simulink library "Suspension"  (R2025b)
settings: Solver=VariableStepAuto  StartTime=0.0  StopTime=10.0  RelTol=1e-3
undefined symbols (not defined in the file): Init, Vehicle
libraries: Susp_AxleTA2PR x1, Susp_AxleTA3 x1, Susp_AxleTA4Watts x1, Susp_LUT x1, Suspension_Linkage x1, Suspension_Linkage_Decoupled x1, Susp_LiveAxle x1, Susp_DOF15 x1, Susp_TwistBeam x1
Description:
  | Component of Simscape Vehicle Templates Library
  | 
  | Copyright 2018-2025 The MathWorks, Inc.
settings Model: Creator=smiller  LastModifiedBy=smiller
settings SolverCC: AlgebraicLoopSolver=TrustRegion
settings DataIOCC: ReturnWorkspaceOutputs=off
settings DebuggingCC: UnconnectedInputMsg=warning  UnconnectedOutputMsg=warning  UnconnectedLineMsg=warning  ArithmeticOperatorsInVariantConditions=warning
settings ModelReferenceCC: EnableRefExpFcnMdlSchedulingChecks=on
settings SFSimCC: CustomCodeUndefinedFunction=UseInterfaceOnly
settings RTWCC: GPUComputeCapability=3.5

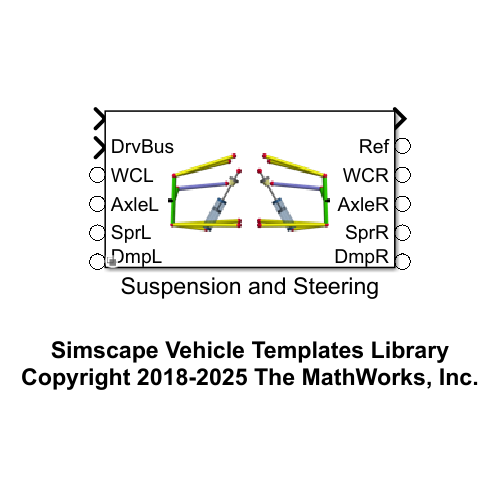
[thumbnail: Simulink's stored preview of the top-level diagram]
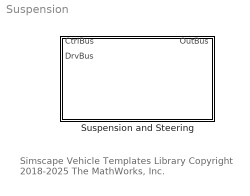
== system Suspension ==
  note: Simscape Vehicle Templates Library
      | Copyright 2018-2025 The MathWorks, Inc.
  Suspension and Steering : Subsystem  Variant=on  VariantControlMode=label  VariantControl=Variant1  LabelModeActiveChoice=Linkage  mask(Suspension and Steering){Susp=Vehicle.Chassis.SuspA1, Init=Init.Axle1, VariantLabel=Vehicle.Chassis.SuspA1.class.Value}
      mask prompts: Susp "Suspension Parameters"; Init "Initial Values"; VariantLabel "Variant Label"
      mask help: Models suspension and optional steering system for one axle. Option is chosen by string provided in Variant Label. The parameters for the selected option are contained in Suspension Parameters data structure.
      mask init:
      | curblk = gcb;
      | 
      | % Set variant for this block 
      | set_param(curblk,'LabelModeActiveChoice',VariantLabel);

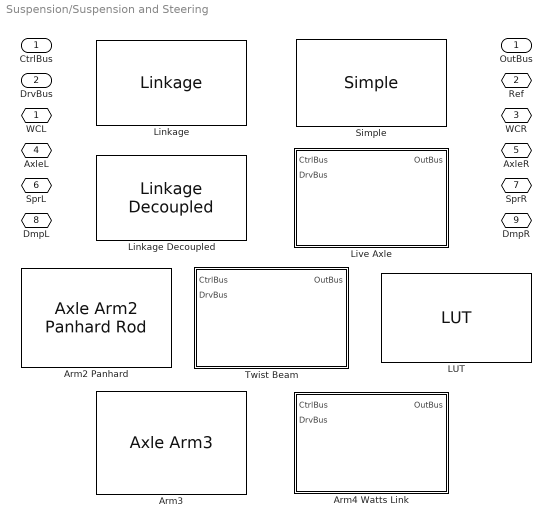
== system Suspension/Suspension and Steering ==
  "CtrlBus " : Inport
  DrvBus : Inport  Port=2
  Arm2 Panhard : Susp_AxleTA2PR/Axle Arm2 Panhard Rod  VariantControl=AxleTA2PR  Init=Init  Susp=Susp
  Arm3 : Susp_AxleTA3/Axle Arm3  VariantControl=AxleTA3  Init=Init  Susp=Susp
  Arm4 Watts Link : Subsystem  VariantControl=AxleTA4Watts  mask{Susp=Vehicle.Chassis.SuspA2}
      mask prompts: Susp "Axle 4 Trailing Arm, Watts Link (structure)"
      mask Display: image('sm_car_vehicle_susp_axleta4watts_IMAGE.png');
  LUT : Susp_LUT/LUT  SystemSampleTime=-1  VariantControl=LUT  VariantActivationTime=update diagram  Latency=0  AutoFrameSizeCalculation=off
  Linkage : Suspension_Linkage/Linkage  VariantControl=Linkage
  Linkage Decoupled : Suspension_Linkage_Decoupled/Linkage Decoupled  VariantControl=Decoupled
  Live Axle : Subsystem  VariantControl=LiveAxle  mask(Live Axle){LiveAxle=Susp.LiveAxle}
      mask prompts: LiveAxle "Live Axle (structure)"
      mask help: Models a live axle suspension with no steering.
      mask Display: image('sm_car_vehicle_susp_liveaxle_IMAGE.png');
  Simple : Susp_DOF15/Simple  VariantControl=Simple
  Twist Beam : Subsystem  VariantControl=TwistBeam  mask{TwistBeam=Susp.TwistBeam}
      mask prompts: TwistBeam "Twist Beam (structure)"
      mask Display: image('sm_car_vehicle_susp_twistbeam_IMAGE.png');
  WCL : PMIOPort  Side=Left
  Ref : PMIOPort  Port=2  Side=Right
  WCR : PMIOPort  Port=3  Side=Right
  AxleL : PMIOPort  Port=4  Side=Left
  AxleR : PMIOPort  Port=5  Side=Right
  SprL : PMIOPort  Port=6  Side=Left
  SprR : PMIOPort  Port=7  Side=Right
  DmpL : PMIOPort  Port=8  Side=Left
  DmpR : PMIOPort  Port=9  Side=Right
  OutBus : Outport  VectorParamsAs1DForOutWhenUnconnected=off

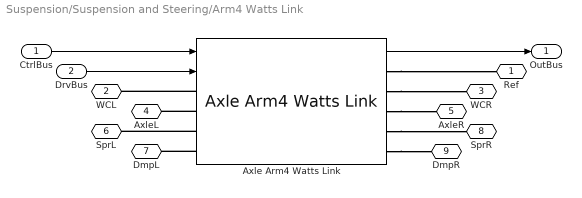
== system Suspension/Suspension and Steering/Arm4 Watts Link ==
  CtrlBus : Inport
  DrvBus : Inport  Port=2
  Axle Arm4 Watts Link : Susp_AxleTA4Watts/Axle Arm4 Watts Link  VariantControl=LiveAxle  Init=Init  hp_damper_top=Susp.AxleTA4Watts.Damper.sTop.Value  hp_damper_bot=Susp.AxleTA4Watts.Damper.sBottom.Value  hp_spring_top=Susp.AxleTA4Watts.Spring.sTop.Value  hp_spring_bot=Susp.AxleTA4Watts.Spring.sBottom.Value  hp_ua_body=Susp.AxleTA4Watts.TrailingArmUpper.sBody.Value  hp_ua_axle=Susp.AxleTA4Watts.TrailingArmUpper.sAxle.Value  hp_la_body=Susp.AxleTA4Watts.TrailingArmLower.sBody.Value  hp_la_axle=Susp.AxleTA4Watts.TrailingArmLower.sAxle.Value  hp_wattsu_body=Susp.AxleTA4Watts.WattsLinkUpper.sBody.Value  hp_wattsu_pivot=Susp.AxleTA4Watts.WattsLinkUpper.sPivot.Value  hp_wattsl_body=Susp.AxleTA4Watts.WattsLinkLower.sBody.Value  hp_wattsl_pivot=Susp.AxleTA4Watts.WattsLinkLower.sPivot.Value  hp_wattsp_axle=Susp.AxleTA4Watts.WattsLinkPivot.sAxle.Value  hp_axle_cg=Susp.AxleTA4Watts.Axle.sCG.Value  hp_whl_ctr=Susp.AxleTA4Watts.Axle.sWheelCentre.Value  hp_chassis_bumpstop=Susp.AxleTA4Watts.Bumpstop.sChassis.Value  hp_axle_bumpstop=Susp.AxleTA4Watts.Bumpstop.sAxle.Value  axle_mass=Susp.AxleTA4Watts.Axle.m.Value  stub_axle_len=Susp.AxleTA4Watts.StubAxle.xAxle.Value  stub_axle_mass=Susp.AxleTA4Watts.StubAxle.m.Value  axle_whlc_to_bearing=Susp.AxleTA4Watts.Axle.xWCtoBearing.Value  ua_mass=Susp.AxleTA4Watts.TrailingArmUpper.m.Value  la_mass=Susp.AxleTA4Watts.TrailingArmLower.m.Value  wattsu_mass=Susp.AxleTA4Watts.WattsLinkUpper.m.Value  wattsl_mass=Susp.AxleTA4Watts.WattsLinkLower.m.Value  wattsp_mass=Susp.AxleTA4Watts.WattsLinkLower.m.Value  clr_conn_rod=Visual.hp.clr  opc_conn_rod=Visual.hp.opc  size_conn_rod=Visual.hp.rad  clr_rod=Visual.UpperArm.clr  opc_rod=Visual.part.opc  radius_rod=Visual.UpperArm.rad  clr_link=Visual.Pushrod.clr  opc_link=Visual.part.opc  radius_link=Visual.Pushrod.rad  axle_clr=Visual.Axle.clr  axle_opc=Visual.part.opc  clr_stub_axle=Visual.Axle.clr  opc_stub_axle=Visual.part.opc  rad_stub_axle=Visual.Axle.rad  shock_pist_mass=Susp.AxleTA4Watts.Damper.mPiston.Value  shock_cyl_mass=Susp.AxleTA4Watts.Damper.mCylinder.Value  shock_xmax=Susp.AxleTA4Watts.Endstop.xMax.Value  shock_xmin=Susp.AxleTA4Watts.Endstop.xMin.Value  spring_mass=Susp.AxleTA4Watts.Spring.m.Value  Bumpstop_Type=Susp.AxleTA4Watts.Bumpstop.class.Value  bumpstop_height=Susp.AxleTA4Watts.Bumpstop.xHeight.Value  bumpstop_k=Susp.AxleTA4Watts.Bumpstop.K.Value  bumpstop_d=Susp.AxleTA4Watts.Bumpstop.d.Value  bumpstop_xTrans=Susp.AxleTA4Watts.Bumpstop.xTransition.Value  bumpstop_ptcld=Susp.AxleTA4Watts.Bumpstop.sPointCloud.Value
  Ref : PMIOPort  Side=Right
  WCL : PMIOPort  Port=2  Side=Left
  WCR : PMIOPort  Port=3  Side=Right
  AxleL : PMIOPort  Port=4  Side=Left
  AxleR : PMIOPort  Port=5  Side=Right
  SprL : PMIOPort  Port=6  Side=Left
  DmpL : PMIOPort  Port=7  Side=Left
  SprR : PMIOPort  Port=8  Side=Right
  DmpR : PMIOPort  Port=9  Side=Right
  OutBus : Outport
  wires:
  Axle Arm4 Watts Link/1 -> OutBus/1
  CtrlBus/1 -> Axle Arm4 Watts Link/1
  DrvBus/1 -> Axle Arm4 Watts Link/2
  connections:
  Axle Arm4 Watts Link/RConn1 -- Ref/RConn1
  Axle Arm4 Watts Link/RConn3 -- AxleR/RConn1
  Axle Arm4 Watts Link/RConn2 -- WCR/RConn1
  Axle Arm4 Watts Link/RConn5 -- DmpR/RConn1
  Axle Arm4 Watts Link/LConn3 -- SprL/RConn1
  Axle Arm4 Watts Link/LConn4 -- DmpL/RConn1
  Axle Arm4 Watts Link/RConn4 -- SprR/RConn1
  Axle Arm4 Watts Link/LConn2 -- AxleL/RConn1
  Axle Arm4 Watts Link/LConn1 -- WCL/RConn1

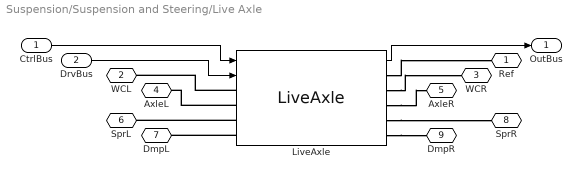
== system Suspension/Suspension and Steering/Live Axle ==
  CtrlBus : Inport
  DrvBus : Inport  Port=2
  LiveAxle : Susp_LiveAxle/LiveAxle  VariantControl=LiveAxle  Init=Init  hp_shock_top=LiveAxle.Shock.sTop.Value  hp_shock_bot=LiveAxle.Shock.sBottom.Value  hp_leaf_body=LiveAxle.Leaf.sBody.Value  hp_leaf_axle=LiveAxle.Leaf.sAxle.Value  hp_whl_ctr=LiveAxle.sWheelCentre.Value  axle_rad=LiveAxle.Axle.radius.Value  axle_mass=LiveAxle.Axle.m.Value  leaf_w=LiveAxle.Leaf.xWidth.Value  leaf_t=LiveAxle.Leaf.xThickness.Value  leaf_rho=LiveAxle.Leaf.density.Value  leaf_E=LiveAxle.Leaf.E.Value  leaf_nu=LiveAxle.Leaf.nu.Value  leaf_zeta=LiveAxle.Leaf.zDamping.Value  piston_mass=LiveAxle.Shock.mPiston.Value  cyl_mass=LiveAxle.Shock.mCylinder.Value  shock_xmax=LiveAxle.Endstop.xMax.Value  shock_xmin=LiveAxle.Endstop.xMin.Value
  Ref : PMIOPort  Side=Right
  WCL : PMIOPort  Port=2  Side=Left
  WCR : PMIOPort  Port=3  Side=Right
  AxleL : PMIOPort  Port=4  Side=Left
  AxleR : PMIOPort  Port=5  Side=Right
  SprL : PMIOPort  Port=6  Side=Left
  DmpL : PMIOPort  Port=7  Side=Left
  SprR : PMIOPort  Port=8  Side=Right
  DmpR : PMIOPort  Port=9  Side=Right
  OutBus : Outport  VectorParamsAs1DForOutWhenUnconnected=off
  wires:
  LiveAxle/1 -> OutBus/1
  CtrlBus/1 -> LiveAxle/1
  DrvBus/1 -> LiveAxle/2
  connections:
  LiveAxle/LConn4 -- DmpL/RConn1
  LiveAxle/LConn3 -- SprL/RConn1
  LiveAxle/RConn3 -- AxleR/RConn1
  LiveAxle/LConn2 -- AxleL/RConn1
  LiveAxle/LConn1 -- WCL/RConn1
  LiveAxle/RConn1 -- Ref/RConn1
  LiveAxle/RConn4 -- SprR/RConn1
  LiveAxle/RConn2 -- WCR/RConn1
  LiveAxle/RConn5 -- DmpR/RConn1

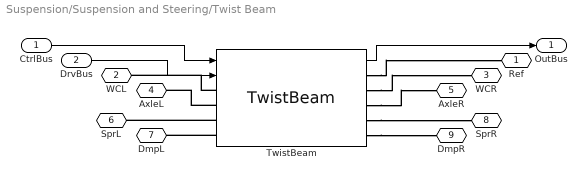
== system Suspension/Suspension and Steering/Twist Beam ==
  CtrlBus : Inport
  DrvBus : Inport  Port=2
  TwistBeam : Susp_TwistBeam/TwistBeam  VariantControl=TwistBeam  Init=Init  hp_arm=TwistBeam.TrailingArm.sBody.Value  hp_dmp_top=TwistBeam.Damper.sTop.Value  hp_dmp_bot=TwistBeam.Damper.sBottom.Value  hp_spr_top=TwistBeam.Spring.sTop.Value  hp_spr_bot=TwistBeam.Spring.sBottom.Value  hp_beam=TwistBeam.Beam.sOutboard.Value  hp_whl_ctr=TwistBeam.TrailingArm.sWheelCentre.Value  Arm_to_Subframe=TwistBeam.Arm_to_Subframe  Damper_to_Subframe=TwistBeam.Damper_to_Subframe  Damper_to_Arm=TwistBeam.Damper_to_Arm  arm_mass=TwistBeam.TrailingArm.m.Value  axle_mass=TwistBeam.TrailingArm.mAxle.Value  axle_len=TwistBeam.TrailingArm.xAxle.Value  axle_whlc_to_bearing=TwistBeam.TrailingArm.xWCtoBearing.Value  beam_rho=TwistBeam.Beam.density.Value  beam_E=TwistBeam.Beam.E.Value  beam_nu=TwistBeam.Beam.nu.Value  beam_zeta=TwistBeam.Beam.zDamping.Value  xc_x=TwistBeam.Beam.xcX.Value  xc_z=TwistBeam.Beam.xcZ.Value  beam_numElements=TwistBeam.Beam.numElements.Value  opc_beam=Visual.part.opc  clr_beam=Visual.clr.orangedark  radius_axle=Visual.Axle.rad  clr_axle=Visual.Axle.clr  opc_axle=Visual.part.opc  clr_upr=Visual.UpperArm.clr  opc_upr=Visual.part.opc  piston_mass=TwistBeam.Damper.mPiston.Value  cyl_mass=TwistBeam.Damper.mCylinder.Value  damper_xmax=TwistBeam.Endstop.xMax.Value  damper_xmin=TwistBeam.Endstop.xMin.Value  spring_mass=TwistBeam.Spring.m.Value
  Ref : PMIOPort  Side=Right
  WCL : PMIOPort  Port=2  Side=Left
  WCR : PMIOPort  Port=3  Side=Right
  AxleL : PMIOPort  Port=4  Side=Left
  AxleR : PMIOPort  Port=5  Side=Right
  SprL : PMIOPort  Port=6  Side=Left
  DmpL : PMIOPort  Port=7  Side=Left
  SprR : PMIOPort  Port=8  Side=Right
  DmpR : PMIOPort  Port=9  Side=Right
  OutBus : Outport
  wires:
  DrvBus/1 -> TwistBeam/2
  CtrlBus/1 -> TwistBeam/1
  TwistBeam/1 -> OutBus/1
  connections:
  TwistBeam/LConn1 -- WCL/RConn1
  TwistBeam/LConn2 -- AxleL/RConn1
  TwistBeam/RConn4 -- SprR/RConn1
  TwistBeam/LConn4 -- DmpL/RConn1
  TwistBeam/LConn3 -- SprL/RConn1
  TwistBeam/RConn5 -- DmpR/RConn1
  TwistBeam/RConn2 -- WCR/RConn1
  TwistBeam/RConn3 -- AxleR/RConn1
  TwistBeam/RConn1 -- Ref/RConn1
